simulink model "parallel_lht_kernel"  (R2019b)
settings: Solver=VariableStepAuto  StartTime=0.0  StopTime=inf  RelTol=1e-3
InitFcn:
  | parallel_lht_setup;
StopFcn:
  | parallel_lht_kernel_compare;
undefined symbols (not defined in the file or in its folder): bt, height, imresize, rgb2gray, width
libraries: hdlsllib x7, simulink x5, dspsrcs4 x1
settings Model: SimulationMode=accelerator  Creator=rgb11127  LastModifiedBy=rgb11127

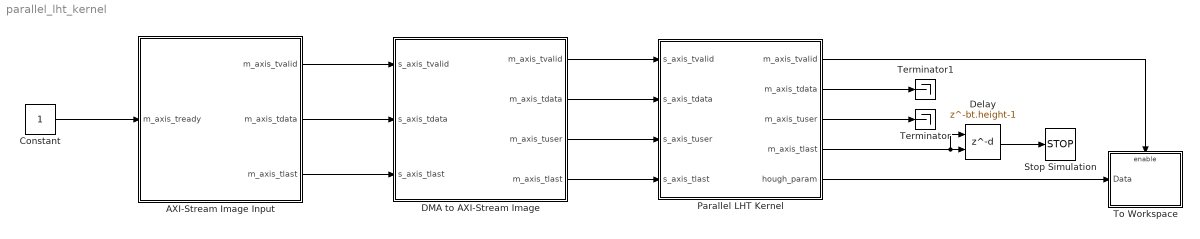
== system parallel_lht_kernel ==
  AXI-Stream Image Input : Subsystem  mask{image=imresize(rgb2gray(imread('peppers.png')), [240, 320]), clk=1/150e6}
      mask prompts: image "Input Image:"; clk "Clock Rate:"
      mask init:
      | [height, width] = size(image);
      mask DialogControl DescGroupVar Prompt: AXI-Stream Image Input
      mask DialogControl DescTextVar Prompt: This block simulates an AXI-Stream image input for interfacing to a hardware accelerator or IP Core.
      mask DialogControl ParameterGroupVar Prompt: Main
  Constant : Constant  OutDataTypeStr=boolean  SampleTime=-1
  DMA to AXI-Stream Image : Subsystem  mask{height=bt.height, width=bt.width, b=1}
      mask prompts: height "Image Height:"; width "Image Width:"; b "Bits"
      mask DialogControl DescGroupVar Prompt: DMA to AXI-Stream Image
      mask DialogControl DescTextVar Prompt: Converts an DMA AXI-Stream packet to the AXI-Stream video standard.
      mask DialogControl Container2 Prompt: Main
  Delay : Delay  DelayLength=bt.height-1  ShowEnablePort=on
      settings: InputPortMap=u0,e6
  Parallel LHT Kernel : Subsystem  mask{height=bt.height, width=bt.width, theta=bt.theta}
      mask prompts: height "Image Height:"; width "Image Width:"; theta "Orientations:"
      mask init:
      | maxRho = ceil(sqrt((height/2)^2+(width/2)^2));
      mask DialogControl ParameterGroupVar Prompt: Main
  Stop Simulation : Stop
  Terminator : Terminator
  Terminator1 : Terminator
  To Workspace : Subsystem  TreatAsAtomicUnit=on
  wires:
  Constant/1 -> AXI-Stream Image Input/1(m_axis_tready)
  AXI-Stream Image Input/1(m_axis_tvalid) -> DMA to AXI-Stream Image/1(s_axis_tvalid)
  AXI-Stream Image Input/2(m_axis_tdata) -> DMA to AXI-Stream Image/2(s_axis_tdata)
  AXI-Stream Image Input/3(m_axis_tlast) -> DMA to AXI-Stream Image/3(s_axis_tlast)
  DMA to AXI-Stream Image/1(m_axis_tvalid) -> Parallel LHT Kernel/1(s_axis_tvalid)
  DMA to AXI-Stream Image/2(m_axis_tdata) -> Parallel LHT Kernel/2(s_axis_tdata)
  DMA to AXI-Stream Image/3(m_axis_tuser) -> Parallel LHT Kernel/3(s_axis_tuser)
  DMA to AXI-Stream Image/4(m_axis_tlast) -> Parallel LHT Kernel/4(s_axis_tlast)
  Parallel LHT Kernel/5(hough_param) -> To Workspace/1(Data)
  Parallel LHT Kernel/1(m_axis_tvalid) -> To Workspace/Enable
  Parallel LHT Kernel/4(m_axis_tlast) -> Delay/1, Delay/2
  Parallel LHT Kernel/3(m_axis_tuser) -> Terminator/1
  Parallel LHT Kernel/2(m_axis_tdata) -> Terminator1/1
  Delay/1 -> Stop Simulation/1

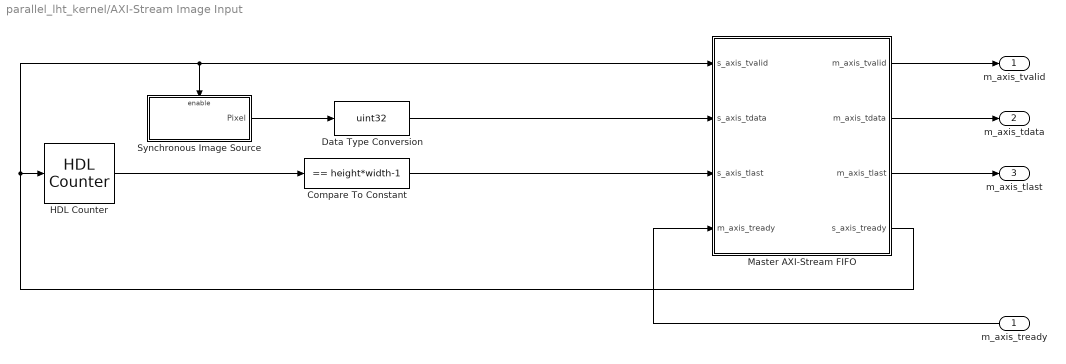
== system parallel_lht_kernel/AXI-Stream Image Input ==
  m_axis_tready : Inport
  Compare To Constant : simulink/Logic and Bit Operations/Compare To Constant  relop===  const=height*width-1  OutDataTypeStr=boolean
  Data Type Conversion : DataTypeConversion  OutDataTypeStr=uint32
  HDL Counter : hdlsllib/Sources/HDL Counter  CountType=Count limited  CountInit=0  CountStep=1  CountMax=width*height-1  CountFromType=Initial value  CountFrom=0  CountResetPort=off  CountLoadPort=off  CountEnbPort=on  CountDirPort=off  CountDataType=Unsigned  CountWordLen=ceil(log2(width*height))  CountFracLen=0  CountSampTime=1
      settings: SourceProductName=Simulink
  Master AXI-Stream FIFO : Subsystem  mask{depth=32}
      mask prompts: depth "FIFO Depth:"
      mask DialogControl DescGroupVar Prompt: Master AXI-Stream FIFO
      mask DialogControl DescTextVar Prompt: A custom AXI-Stream FIFO for interfacing to write channel AXI DMAs.
      mask DialogControl ParameterGroupVar Prompt: Main
  Synchronous Image Source : Subsystem
  m_axis_tvalid : Outport
  m_axis_tdata : Outport  Port=2
  m_axis_tlast : Outport  Port=3
  wires:
  Master AXI-Stream FIFO/2(m_axis_tdata) -> m_axis_tdata/1
  Master AXI-Stream FIFO/3(m_axis_tlast) -> m_axis_tlast/1
  m_axis_tready/1 -> Master AXI-Stream FIFO/4(m_axis_tready)
  Master AXI-Stream FIFO/4(s_axis_tready) -> HDL Counter/1, Master AXI-Stream FIFO/1(s_axis_tvalid), Synchronous Image Source/Enable
  Compare To Constant/1 -> Master AXI-Stream FIFO/3(s_axis_tlast)
  Data Type Conversion/1 -> Master AXI-Stream FIFO/2(s_axis_tdata)
  Master AXI-Stream FIFO/1(m_axis_tvalid) -> m_axis_tvalid/1
  Synchronous Image Source/1(Pixel) -> Data Type Conversion/1
  HDL Counter/1 -> Compare To Constant/1

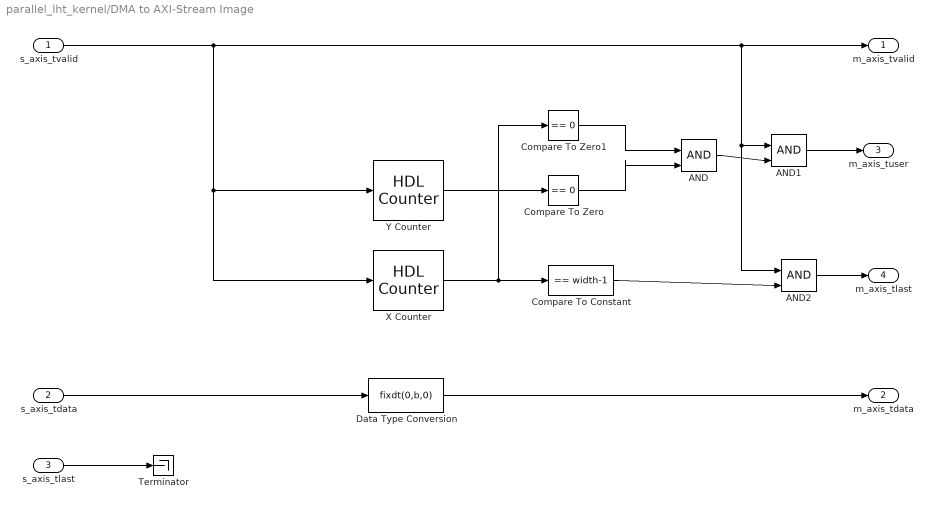
== system parallel_lht_kernel/DMA to AXI-Stream Image ==
  s_axis_tvalid : Inport
  s_axis_tdata : Inport  Port=2
  s_axis_tlast : Inport  Port=3
  AND : Logic  IconShape=distinctive  AllPortsSameDT=off  OutDataTypeStr=boolean
  AND1 : Logic  IconShape=distinctive  AllPortsSameDT=off  OutDataTypeStr=boolean
  AND2 : Logic  IconShape=distinctive  AllPortsSameDT=off  OutDataTypeStr=boolean
  Compare To Constant : simulink/Logic and Bit Operations/Compare To Constant  relop===  const=width-1  OutDataTypeStr=boolean
  Compare To Zero : simulink/Logic and Bit Operations/Compare To Zero  relop===  OutDataTypeStr=boolean
  Compare To Zero1 : simulink/Logic and Bit Operations/Compare To Zero  relop===  OutDataTypeStr=boolean
  Data Type Conversion : DataTypeConversion  OutDataTypeStr=fixdt(0,b,0)  ConvertRealWorld=Stored Integer (SI)
  Terminator : Terminator
  X Counter : hdlsllib/Sources/HDL Counter  CountType=Count limited  CountInit=0  CountStep=1  CountMax=width-1  CountFromType=Initial value  CountFrom=0  CountResetPort=off  CountLoadPort=off  CountEnbPort=on  CountDirPort=off  CountDataType=Unsigned  CountWordLen=ceil(log2(width))  CountFracLen=0  CountSampTime=1
      settings: SourceProductName=Simulink
  Y Counter : hdlsllib/Sources/HDL Counter  CountType=Count limited  CountInit=0  CountStep=1  CountMax=height-1  CountFromType=Initial value  CountFrom=0  CountResetPort=off  CountLoadPort=off  CountEnbPort=on  CountDirPort=off  CountDataType=Unsigned  CountWordLen=ceil(log2(height))  CountFracLen=0  CountSampTime=1
      settings: SourceProductName=Simulink
  m_axis_tvalid : Outport
  m_axis_tdata : Outport  Port=2
  m_axis_tuser : Outport  Port=3
  m_axis_tlast : Outport  Port=4
  wires:
  AND2/1 -> m_axis_tlast/1
  Compare To Constant/1 -> AND2/2
  AND1/1 -> m_axis_tuser/1
  AND/1 -> AND1/2
  s_axis_tlast/1 -> Terminator/1
  s_axis_tdata/1 -> Data Type Conversion/1
  Compare To Zero/1 -> AND/2
  Compare To Zero1/1 -> AND/1
  Y Counter/1 -> Compare To Zero/1
  X Counter/1 -> Compare To Constant/1, Compare To Zero1/1
  s_axis_tvalid/1 -> m_axis_tvalid/1, AND1/1, AND2/1, Y Counter/1, X Counter/1
  Data Type Conversion/1 -> m_axis_tdata/1

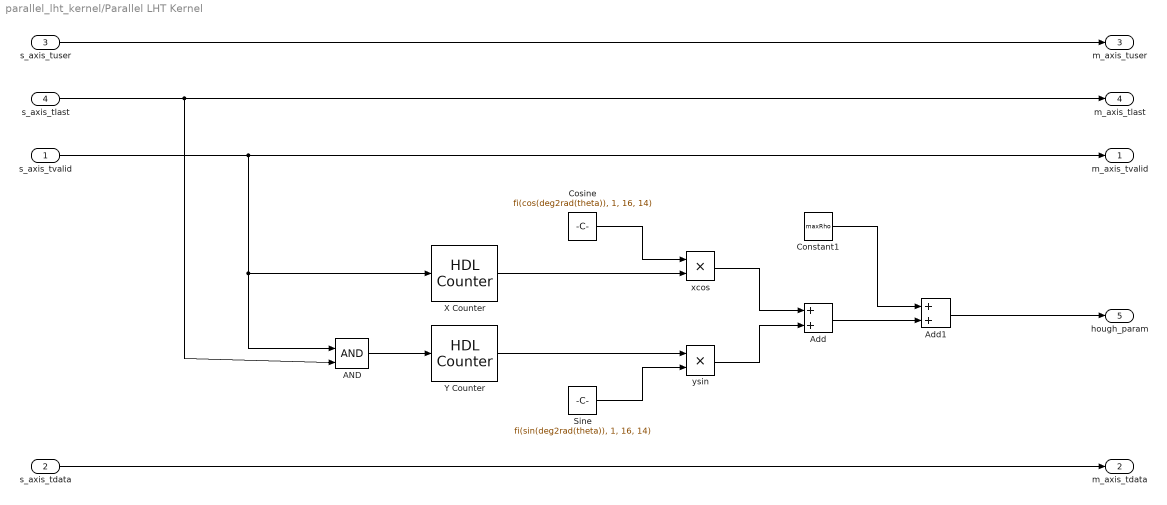
== system parallel_lht_kernel/Parallel LHT Kernel ==
  s_axis_tvalid : Inport
  s_axis_tdata : Inport  Port=2
  s_axis_tuser : Inport  Port=3
  s_axis_tlast : Inport  Port=4
  AND : Logic  IconShape=distinctive  AllPortsSameDT=off  OutDataTypeStr=boolean
  Add : Sum  OutDataTypeStr=fixdt(1,ceil(log2(maxRho*2+1)),0)  RndMeth=Round
  Add1 : Sum  OutDataTypeStr=fixdt(0, ceil(log2(2*maxRho+1)), 0);  RndMeth=Round
  Constant1 : Constant  Value=maxRho  OutDataTypeStr=fixdt(0, ceil(log2(maxRho + 1)), 0);  SampleTime=-1
  Cosine : Constant  Value=fi(cos(deg2rad(theta)), 1, 16, 14)  VectorParams1D=off  OutDataTypeStr=fixdt(1,16,14)  SampleTime=-1
  Sine : Constant  Value=fi(sin(deg2rad(theta)), 1, 16, 14)  VectorParams1D=off  OutDataTypeStr=fixdt(1,16,14)  SampleTime=-1
  X Counter : hdlsllib/Sources/HDL Counter  CountType=Count limited  CountInit=-width/2  CountStep=1  CountMax=width/2-1  CountFromType=Initial value  CountFrom=-width/2  CountResetPort=off  CountLoadPort=off  CountEnbPort=on  CountDirPort=off  CountDataType=Signed  CountWordLen=ceil(log2(width))  CountFracLen=0  CountSampTime=1
      settings: SourceProductName=Simulink
  Y Counter : hdlsllib/Sources/HDL Counter  CountType=Count limited  CountInit=-height/2  CountStep=1  CountMax=height/2-1  CountFromType=Initial value  CountFrom=-height/2  CountResetPort=off  CountLoadPort=off  CountEnbPort=on  CountDirPort=off  CountDataType=Signed  CountWordLen=ceil(log2(height))  CountFracLen=0  CountSampTime=1
      settings: SourceProductName=Simulink
  xcos : Product  OutDataTypeStr=fixdt(1, ceil(log2(width)), 0)  RndMeth=Round
  ysin : Product  OutDataTypeStr=fixdt(1, ceil(log2(height)), 0)  RndMeth=Round
  m_axis_tvalid : Outport
  m_axis_tdata : Outport  Port=2
  m_axis_tuser : Outport  Port=3
  m_axis_tlast : Outport  Port=4
  hough_param : Outport  Port=5
  wires:
  ysin/1 -> Add/2
  s_axis_tvalid/1 -> X Counter/1, AND/1, m_axis_tvalid/1
  AND/1 -> Y Counter/1
  Cosine/1 -> xcos/1
  Y Counter/1 -> ysin/1
  Add/1 -> Add1/2
  xcos/1 -> Add/1
  X Counter/1 -> xcos/2
  Constant1/1 -> Add1/1
  Sine/1 -> ysin/2
  s_axis_tlast/1 -> AND/2, m_axis_tlast/1
  Add1/1 -> hough_param/1
  s_axis_tdata/1 -> m_axis_tdata/1
  s_axis_tuser/1 -> m_axis_tuser/1

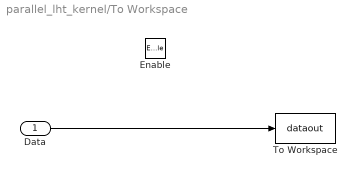
== system parallel_lht_kernel/To Workspace ==
  Data : Inport
  Enable : EnablePort
  To Workspace : ToWorkspace  VariableName=dataout  SampleTime=-1
      settings: Save2DSignal=2-D array (concatenate along first dimension)
  wires:
  Data/1 -> To Workspace/1

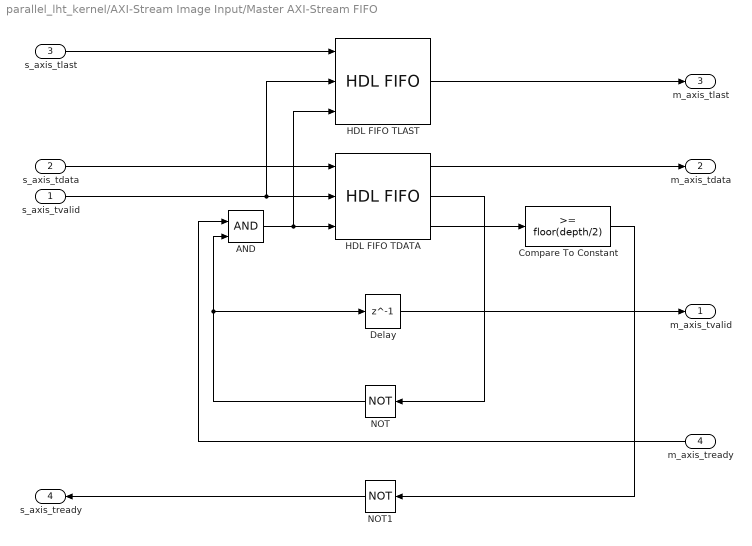
== system parallel_lht_kernel/AXI-Stream Image Input/Master AXI-Stream FIFO ==
  s_axis_tvalid : Inport
  s_axis_tdata : Inport  Port=2
  s_axis_tlast : Inport  Port=3
  m_axis_tready : Inport  Port=4
  AND : Logic  IconShape=distinctive  AllPortsSameDT=off  OutDataTypeStr=boolean
  "Compare To Constant " : simulink/Logic and Bit Operations/Compare To Constant  relop=>=  const=floor(depth/2)  OutDataTypeStr=boolean
  Delay : Delay  DelayLength=1
  HDL FIFO TDATA : hdlsllib/HDL RAMs/HDL FIFO  fifo_size=depth  mode=Classic  ratio=1  push_msg=Error  pop_msg=Error  show_empty=on  show_full=off  show_num=on  LabelModeActiveChoice_Mode=Classic
      settings: SourceProductName=Simulink  SourceProductBaseCode=SL
  HDL FIFO TLAST : hdlsllib/HDL RAMs/HDL FIFO  fifo_size=depth  mode=Classic  ratio=1  push_msg=Error  pop_msg=Error  show_empty=off  show_full=off  show_num=off  LabelModeActiveChoice_Mode=Classic
      settings: SourceProductName=Simulink  SourceProductBaseCode=SL
  NOT : Logic  Operator=NOT  IconShape=distinctive  AllPortsSameDT=off  OutDataTypeStr=boolean
  NOT1 : Logic  Operator=NOT  IconShape=distinctive  AllPortsSameDT=off  OutDataTypeStr=boolean
  m_axis_tvalid : Outport  VectorParamsAs1DForOutWhenUnconnected=off
  m_axis_tdata : Outport  Port=2  VectorParamsAs1DForOutWhenUnconnected=off
  m_axis_tlast : Outport  Port=3  VectorParamsAs1DForOutWhenUnconnected=off
  s_axis_tready : Outport  Port=4
  wires:
  Delay/1 -> m_axis_tvalid/1
  s_axis_tvalid/1 -> HDL FIFO TDATA/2, HDL FIFO TLAST/2
  s_axis_tdata/1 -> HDL FIFO TDATA/1
  s_axis_tlast/1 -> HDL FIFO TLAST/1
  "Compare To Constant "/1 -> NOT1/1
  NOT1/1 -> s_axis_tready/1
  HDL FIFO TDATA/3 -> "Compare To Constant "/1
  m_axis_tready/1 -> AND/1
  NOT/1 -> AND/2, Delay/1
  AND/1 -> HDL FIFO TDATA/3, HDL FIFO TLAST/3
  HDL FIFO TDATA/2 -> NOT/1
  HDL FIFO TLAST/1 -> m_axis_tlast/1
  HDL FIFO TDATA/1 -> m_axis_tdata/1

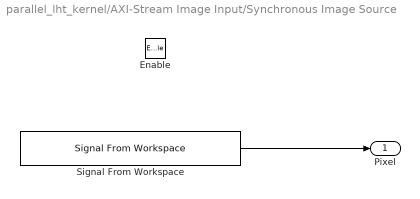
== system parallel_lht_kernel/AXI-Stream Image Input/Synchronous Image Source ==
  Enable : EnablePort
  Signal From Workspace : dspsrcs4/Signal From Workspace  X=reshape(image', [height*width, 1])  Ts=clk  nsamps=1  OutputAfterFinalValue=Cyclic repetition  ignoreOrWarnInputAndFrameLengths=off  OutputFrames=off
  Pixel : Outport
  wires:
  Signal From Workspace/1 -> Pixel/1
